simulink model "PowerLimiterModel"  (R2024b)
settings: Solver=VariableStepAuto  StartTime=0.0  StopTime=20  RelTol=1e-3

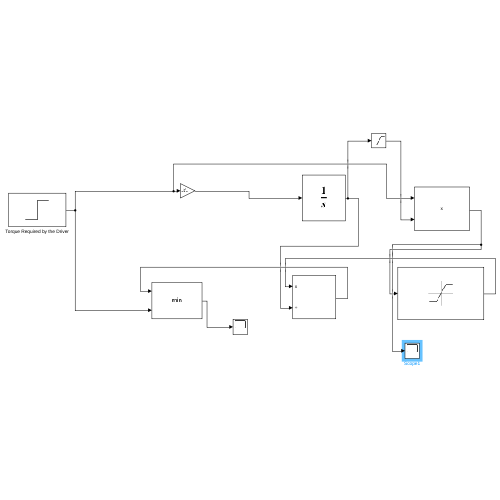
[thumbnail: Simulink's stored preview of the top-level diagram]
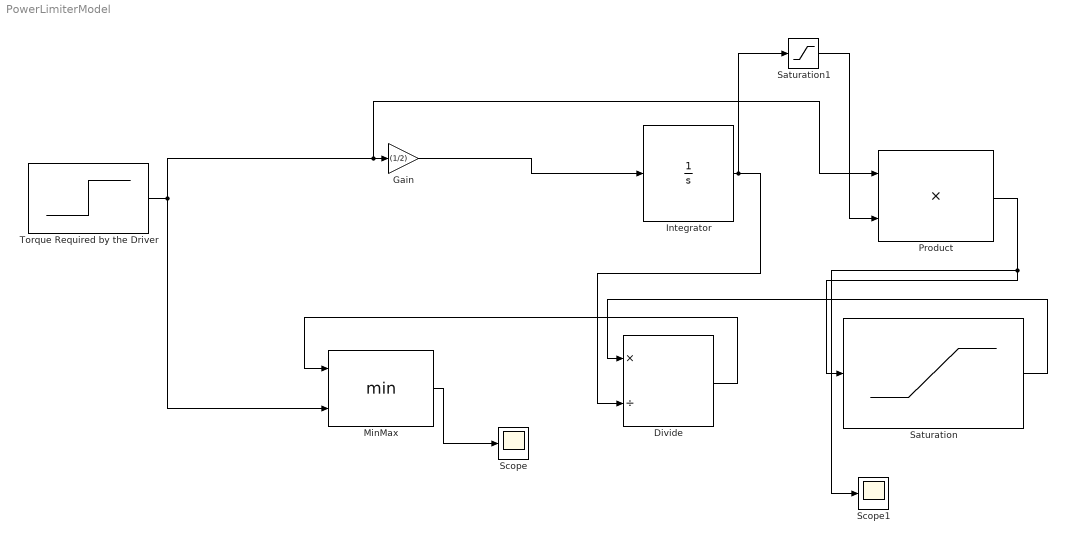
== system PowerLimiterModel ==
  Divide : Product  Inputs=*/
  Gain : Gain  Gain=(1/2)
  Integrator : Integrator
  MinMax : MinMax  Inputs=2
  Product : Product
  Saturation : Saturate  UpperLimit=80000  LowerLimit=0
  Saturation1 : Saturate  UpperLimit=800  LowerLimit=0.1
  Scope : Scope
  Scope1 : Scope
  Torque Required by the Driver : Step  After=100  SampleTime=0
  wires:
  Product/1 -> Scope1/1, Saturation/1
  Saturation/1 -> Divide/1
  Divide/1 -> MinMax/1
  MinMax/1 -> Scope/1
  Integrator/1 -> Saturation1/1, Divide/2
  Torque Required by the Driver/1 -> Product/1, Gain/1, MinMax/2
  Gain/1 -> Integrator/1
  Saturation1/1 -> Product/2
